simulink model "StateTransitionTable_test1"  (R2017a)
settings: Solver=VariableStepAuto  StartTime=0.0  StopTime=inf  RelTol=1e-3
libraries: simulink x1
settings Model: Creator=nishito  LastModifiedBy=nishito

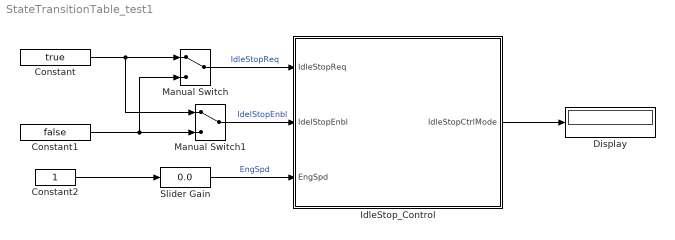
== system StateTransitionTable_test1 ==
  Constant : Constant  Value=true
  Constant1 : Constant  Value=false
  Constant2 : Constant
  Display : Display
  IdleStop_Control : Subsystem
  Manual Switch : ManualSwitch
  Manual Switch1 : ManualSwitch
  Slider Gain : simulink/Math Operations/Slider Gain  gain=0.0  low=0  high=600
  wires:
  Constant2/1 -> Slider Gain/1
  Constant/1 -> Manual Switch1/1, Manual Switch/1
  Constant1/1 -> Manual Switch/2, Manual Switch1/2
  Manual Switch/1 -> IdleStop_Control/1(IdleStopReq)  "IdleStopReq"
  Manual Switch1/1 -> IdleStop_Control/2(IdelStopEnbl)  "IdelStopEnbl"
  Slider Gain/1 -> IdleStop_Control/3(EngSpd)  "EngSpd"
  IdleStop_Control/1(IdleStopCtrlMode) -> Display/1

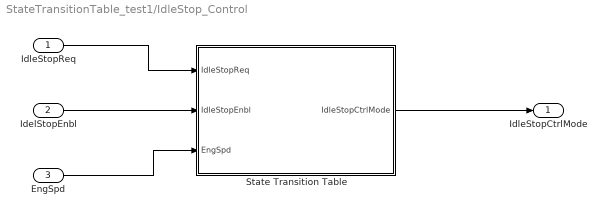
== system StateTransitionTable_test1/IdleStop_Control ==
  IdleStopReq : Inport
  IdelStopEnbl : Inport  Port=2
  EngSpd : Inport  Port=3
  State Transition Table : State Transition Table  TreatAsAtomicUnit=on
  IdleStopCtrlMode : Outport
  wires:
  EngSpd/1 -> State Transition Table/3(EngSpd)
  IdleStopReq/1 -> State Transition Table/1(IdleStopReq)
  IdelStopEnbl/1 -> State Transition Table/2(IdleStopEnbl)
  State Transition Table/1(IdleStopCtrlMode) -> IdleStopCtrlMode/1

== stateflow chart StateTransitionTable_test1/IdleStop_Control/State Transition Table ==
  state EngineStop
    en:
    IdleStopCtrlMode=0;
  state IdleStop
    en:
    IdleStopCtrlMode=1;
  state EngineStart
    en:
    IdleStopCtrlMode=2;
  state IdleStopWait
    en:
    IdleStopCtrlMode=3;
  state IdleStopPrepare
    en:
    IdleStopCtrlMode=4;
  state EngineRun
    en:
    IdleStopCtrlMode=5;
  (default) -> EngineStop
  (junction 32) -> EngineStop
  (junction 52) -> (junction 32)
  EngineStop -> (junction 70) : [EngSpd>300]% Engine run cond
  (junction 70) -> (junction 28)
  (junction 65) -> IdleStop
  (junction 67) -> (junction 65)
  IdleStop -> EngineStart : [~IdleStopReq]% IdleStop end cond.
  EngineStart -> IdleStop [order 2] : [IdleStopReq]% IdleStop restart cond.
  EngineStart -> (junction 28) [order 1] : [EngSpd>300]% Engine run cond
  (junction 28) -> (junction 26)
  IdleStopWait -> (junction 67) [order 1] : [EngSpd<50]% IdlaStopStartCond.
  IdleStopWait -> IdleStopPrepare [order 2] : [~IdleStopEnbl || ~IdleStopReq]% IdleStop cancel cond.
  IdleStopPrepare -> IdleStopWait [order 1] : [IdleStopEnbl]% IdleStop wait cond.
  IdleStopPrepare -> (junction 52) [order 3] : [EngSpd<50]% Engine stop cond.
  (junction 48) -> (junction 52)
  IdleStopPrepare -> EngineRun [order 2] : [~IdleStopReq]% IdleStop cancel cond.
  EngineRun -> IdleStopPrepare [order 1] : [IdleStopReq]% IdleStop prepare cond.
  EngineRun -> (junction 48) [order 2] : [EngSpd<50]% Engine stop cond.
  (junction 26) -> EngineRun
  data: IdleStopReq input; IdleStopEnbl input; EngSpd input; IdleStopCtrlMode output
